simulink model "profilazione_legacy"  (R2023b)
settings: Solver=FixedStepDiscrete  StartTime=0.0  StopTime=60  FixedStep=1/250  RelTol=1e-3
values from neighbouring files (symbols this model uses):
  amplitude_1 = 20e-6    (= 2e-05)    [STUBSCRIPT.m]    (also in main.m; main_calibrazione.m; profilazione.m; setup.m)
  amplitude_2 = 30e-6    (= 3e-05)    [STUBSCRIPT.m]    (also in main.m; main_calibrazione.m; profilazione.m; setup.m)
  amplitude_3 = 40e-6    (= 4e-05)    [STUBSCRIPT.m]    (also in main.m; main_calibrazione.m; profilazione.m; setup.m)
  amplitude_4 = 50e-6    (= 5e-05)    [STUBSCRIPT.m]    (also in main.m; main_calibrazione.m; profilazione.m; setup.m)
  unicorn_f = 250    [STUBSCRIPT.m]    (also in main.m; main_calibrazione.m; profilazione.m)
undefined symbols (not defined in the file or in its folder): UN
libraries: simulink x8, dspfdesign x7, UnicornLib x1
settings Model: Creator=Utente  LastModifiedBy=moggi
settings DebuggingCC: UnconnectedInputMsg=warning  UnconnectedOutputMsg=warning  UnconnectedLineMsg=warning
settings ModelReferenceCC: EnableRefExpFcnMdlSchedulingChecks=on
settings RTWCC: DLArmComputeVersion=19.05
settings ConfigComp: CovBoundaryAbsTol=1.0e-5

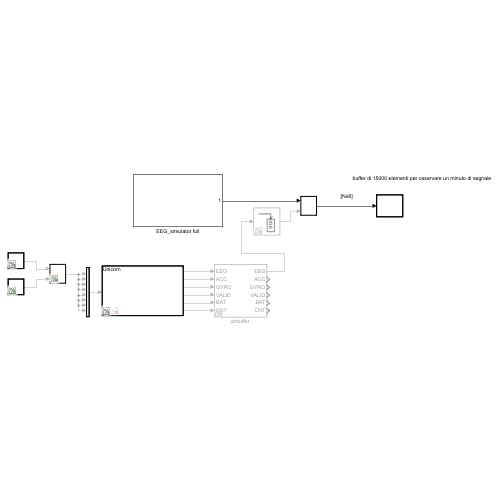
[thumbnail: Simulink's stored preview of the top-level diagram]
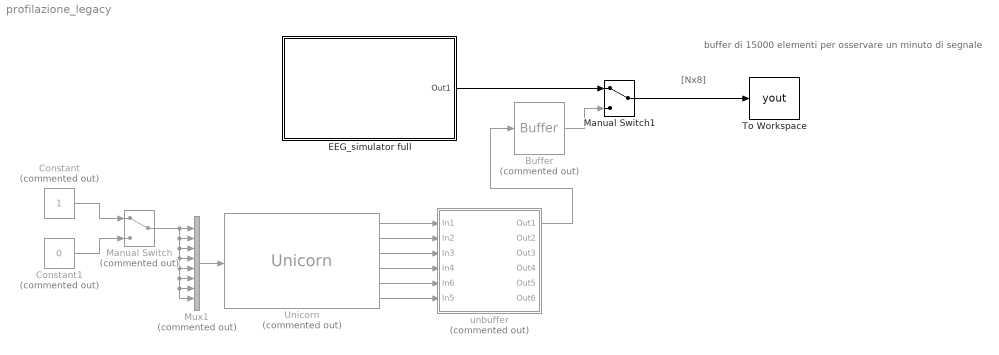
== system profilazione_legacy ==
  note: buffer di 15000 elementi per osservare un minuto di segnale
  note: [Nx8]
  Buffer : Buffer  Commented=on  N=15000  OutputFrames=off
  Constant : Constant  Commented=on  OutDataTypeStr=boolean
  Constant1 : Constant  Commented=on  Value=0  OutDataTypeStr=boolean
  EEG_simulator full : Subsystem
  Manual Switch : ManualSwitch  Commented=on
  Manual Switch1 : ManualSwitch
  Mux1 : Mux  Commented=on  Inputs=8
  To Workspace : ToWorkspace  VariableName=yout  SampleTime=-1
      settings: Save2DSignal=2-D array (concatenate along first dimension)
  Unicorn : UnicornLib/Unicorn  Commented=on  serial=UN-2023.04.40  old_serial=UN-2023.04.40  frame_length=1  input_source=Electrode
      settings: SourceProductName=Unicorn
  "unbuffer " : Subsystem  Commented=on
      mask Display:
      | port_label('input',1,'EEG')
      | port_label('input',2,'ACC')
      | port_label('input',3,'GYRO')
      | port_label('input',4,'VALID')
      | port_label('input',5,'BAT')
      | port_label('input',6,'CNT')
      | port_label('output',1,'EEG')
      | port_label('output',2,'ACC')
      | port_label('output',3,'GYRO')
      | port_label('output',4,'VALID')
      | port_label('output',5,'BAT')
      | port_label('output',6,'CNT')
  wires:
  Constant/1 -> Manual Switch/1
  Mux1/1 -> Unicorn/1
  Manual Switch/1 -> Mux1/8, Mux1/7, Mux1/6, Mux1/5, Mux1/4, Mux1/3, Mux1/2, Mux1/1
  Constant1/1 -> Manual Switch/2
  EEG_simulator full/1(Out1) -> Manual Switch1/1
  Unicorn/1 -> "unbuffer "/1(In1)
  Unicorn/2 -> "unbuffer "/2(In2)
  Unicorn/3 -> "unbuffer "/3(In3)
  Unicorn/4 -> "unbuffer "/4(In4)
  Unicorn/5 -> "unbuffer "/5(In6)
  Unicorn/6 -> "unbuffer "/6(In5)
  "unbuffer "/1(Out1) -> Buffer/1
  Buffer/1 -> Manual Switch1/2
  Manual Switch1/1 -> To Workspace/1

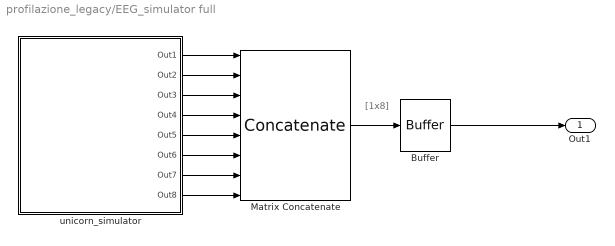
== system profilazione_legacy/EEG_simulator full ==
  note: [1x8]
  Buffer : Buffer  N=15000  OutputFrames=off
  Matrix Concatenate : Concatenate  NumInputs=8  Mode=Multidimensional array  ConcatenateDimension=2
  unicorn_simulator : Subsystem
  Out1 : Outport
  wires:
  unicorn_simulator/1(Out1) -> Matrix Concatenate/1
  unicorn_simulator/2(Out2) -> Matrix Concatenate/2
  Matrix Concatenate/1 -> Buffer/1
  unicorn_simulator/8(Out8) -> Matrix Concatenate/8
  unicorn_simulator/7(Out7) -> Matrix Concatenate/7
  unicorn_simulator/6(Out6) -> Matrix Concatenate/6
  unicorn_simulator/5(Out5) -> Matrix Concatenate/5
  unicorn_simulator/4(Out4) -> Matrix Concatenate/4
  unicorn_simulator/3(Out3) -> Matrix Concatenate/3
  Buffer/1 -> Out1/1

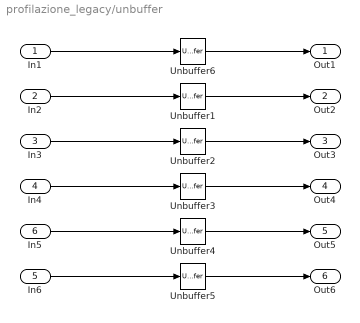
== system profilazione_legacy/unbuffer  ==
  In1 : Inport
  In2 : Inport  Port=2
  In3 : Inport  Port=3
  In4 : Inport  Port=4
  In6 : Inport  Port=5
  In5 : Inport  Port=6
  Unbuffer{1..6} (6 alike) : Unbuffer
  Out1 : Outport
  Out2 : Outport  Port=2
  Out3 : Outport  Port=3
  Out4 : Outport  Port=4
  Out5 : Outport  Port=5
  Out6 : Outport  Port=6
  wires:
  In1/1 -> Unbuffer6/1
  In6/1 -> Unbuffer5/1
  In2/1 -> Unbuffer1/1
  In3/1 -> Unbuffer2/1
  In4/1 -> Unbuffer3/1
  In5/1 -> Unbuffer4/1
  Unbuffer4/1 -> Out5/1
  Unbuffer5/1 -> Out6/1
  Unbuffer3/1 -> Out4/1
  Unbuffer2/1 -> Out3/1
  Unbuffer1/1 -> Out2/1
  Unbuffer6/1 -> Out1/1

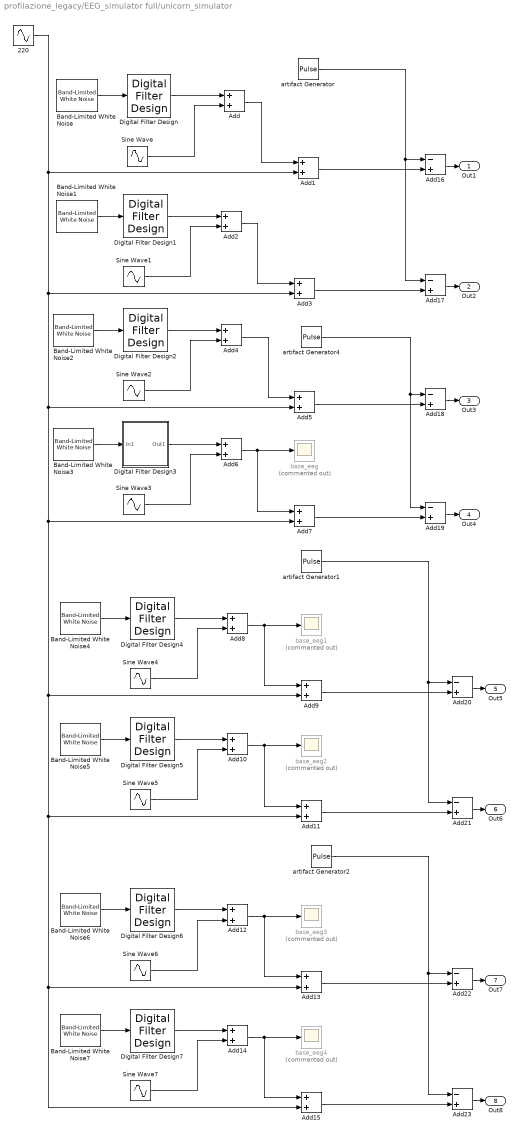
== system profilazione_legacy/EEG_simulator full/unicorn_simulator ==
  220 : Sin  SineType=Sample based  Amplitude=12e-6  Frequency=314.15  SampleTime=1/unicorn_f
  Add{,1..15} (16 alike) : Sum
  Add{16..23} (8 alike) : Sum  Inputs=-+
  Band-Limited White Noise : simulink/Sources/Band-Limited White Noise  Cov=[0.00001]  Ts=1/unicorn_f  seed=[23344]
  Band-Limited White Noise1 : simulink/Sources/Band-Limited White Noise  Cov=[0.00001]  Ts=1/unicorn_f  seed=[23344]
  Band-Limited White Noise2 : simulink/Sources/Band-Limited White Noise  Cov=[0.00001]  Ts=1/unicorn_f  seed=[23343]
  Band-Limited White Noise3 : simulink/Sources/Band-Limited White Noise  Cov=[0.00001]  Ts=1/unicorn_f  seed=[23343]
  Band-Limited White Noise4 : simulink/Sources/Band-Limited White Noise  Cov=[0.00001]  Ts=1/unicorn_f  seed=[23342]
  Band-Limited White Noise5 : simulink/Sources/Band-Limited White Noise  Cov=[0.00001]  Ts=1/unicorn_f  seed=[23342]
  Band-Limited White Noise6 : simulink/Sources/Band-Limited White Noise  Cov=[0.00001]  Ts=1/unicorn_f  seed=[23341]
  Band-Limited White Noise7 : simulink/Sources/Band-Limited White Noise  Cov=[0.00001]  Ts=1/unicorn_f  seed=[23341]
  Digital Filter Design{,1..2,4..7} (7 alike) : dspfdesign/Digital Filter Design  mwdsp_browser_bugfix_var=off
  Digital Filter Design3 : Subsystem  Description=Replaced Block  mask(Replaced Block){}
      mask help: This block has been replaced with an empty subsystem because it used functionality that is unavailable in Simulink R2023b.
      mask Display: fprintf('Replaced: %s\n','Digital Filter Design')
  Sine Wave : Sin  SineType=Sample based  Amplitude=amplitude_1  Frequency=62.83  SampleTime=1/unicorn_f
  Sine Wave1 : Sin  SineType=Sample based  Amplitude=amplitude_1  Frequency=62.83  SampleTime=1/unicorn_f
  Sine Wave2 : Sin  SineType=Sample based  Amplitude=amplitude_2  Frequency=62.83  SampleTime=1/unicorn_f
  Sine Wave3 : Sin  Amplitude=amplitude_2  Frequency=62.83  SampleTime=1/unicorn_f
  Sine Wave4 : Sin  SineType=Sample based  Amplitude=amplitude_3  Frequency=62.83  SampleTime=1/unicorn_f
  Sine Wave5 : Sin  SineType=Sample based  Amplitude=amplitude_3  Frequency=62.83  SampleTime=1/unicorn_f
  Sine Wave6 : Sin  SineType=Sample based  Amplitude=amplitude_4  Frequency=62.83  SampleTime=1/unicorn_f
  Sine Wave7 : Sin  SineType=Sample based  Amplitude=amplitude_4  Frequency=62.83  SampleTime=1/unicorn_f
  artifact Generator : DiscretePulseGenerator  Amplitude=1000*amplitude_1  Period=25000*(1/unicorn_f)  PulseWidth=30  SampleTime=1/unicorn_f
  artifact Generator1 : DiscretePulseGenerator  Amplitude=1000*amplitude_3  Period=25000*(1/unicorn_f)  PulseWidth=30  SampleTime=1/unicorn_f
  artifact Generator2 : DiscretePulseGenerator  Amplitude=1000*amplitude_4  Period=25000*(1/unicorn_f)  PulseWidth=30  SampleTime=1/unicorn_f
  artifact Generator4 : DiscretePulseGenerator  Amplitude=1000*amplitude_2  Period=25000*(1/unicorn_f)  PulseWidth=30  SampleTime=1/unicorn_f
  base_eeg{,1..4} (5 alike) : Scope  Commented=on
  Out1 : Outport
  Out2 : Outport  Port=2
  Out3 : Outport  Port=3
  Out4 : Outport  Port=4
  Out5 : Outport  Port=5
  Out6 : Outport  Port=6
  Out7 : Outport  Port=7
  Out8 : Outport  Port=8
  wires:
  Add1/1 -> Add16/2
  Sine Wave/1 -> Add/2
  Add/1 -> Add1/1
  220/1 -> Add15/2, Add13/2, Add11/2, Add9/2, Add7/2, Add5/2, Add3/2, Add1/2
  Add5/1 -> Add18/2
  Add18/1 -> Out3/1
  Add20/1 -> Out5/1
  artifact Generator4/1 -> Add19/1, Add18/1
  Sine Wave1/1 -> Add2/2
  Sine Wave3/1 -> Add6/2
  Add9/1 -> Add20/2
  Add16/1 -> Out1/1
  Add7/1 -> Add19/2
  Add13/1 -> Add22/2
  Add8/1 -> Add9/1, base_eeg1/1
  Add15/1 -> Add23/2
  artifact Generator2/1 -> Add22/1, Add23/1
  Add2/1 -> Add3/1
  Add6/1 -> Add7/1, base_eeg/1
  Add4/1 -> Add5/1
  artifact Generator1/1 -> Add21/1, Add20/1
  Add12/1 -> Add13/1, base_eeg3/1
  artifact Generator/1 -> Add16/1, Add17/1
  Add3/1 -> Add17/2
  Add14/1 -> Add15/1, base_eeg4/1
  Add11/1 -> Add21/2
  Sine Wave2/1 -> Add4/2
  Sine Wave7/1 -> Add14/2
  Sine Wave4/1 -> Add8/2
  Sine Wave5/1 -> Add10/2
  Sine Wave6/1 -> Add12/2
  Add10/1 -> Add11/1, base_eeg2/1
  Add22/1 -> Out7/1
  Add19/1 -> Out4/1
  Add23/1 -> Out8/1
  Add17/1 -> Out2/1
  Add21/1 -> Out6/1
  Band-Limited White Noise/1 -> Digital Filter Design/1
  Digital Filter Design/1 -> Add/1
  Band-Limited White Noise1/1 -> Digital Filter Design1/1
  Digital Filter Design1/1 -> Add2/1
  Band-Limited White Noise2/1 -> Digital Filter Design2/1
  Digital Filter Design2/1 -> Add4/1
  Band-Limited White Noise3/1 -> Digital Filter Design3/1(In1)
  Digital Filter Design3/1(Out1) -> Add6/1
  Band-Limited White Noise4/1 -> Digital Filter Design4/1
  Digital Filter Design4/1 -> Add8/1
  Band-Limited White Noise5/1 -> Digital Filter Design5/1
  Digital Filter Design5/1 -> Add10/1
  Band-Limited White Noise6/1 -> Digital Filter Design6/1
  Digital Filter Design6/1 -> Add12/1
  Band-Limited White Noise7/1 -> Digital Filter Design7/1
  Digital Filter Design7/1 -> Add14/1

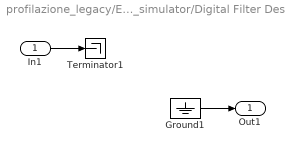
== system profilazione_legacy/EEG_simulator full/unicorn_simulator/Digital Filter Design3 ==
  In1 : Inport
  Ground1 : Ground
  Terminator1 : Terminator
  Out1 : Outport
  wires:
  Ground1/1 -> Out1/1
  In1/1 -> Terminator1/1
